simulink model "online_fuzz_clus"  (Simulink 7.7)
settings: Solver=ode4  StartTime=0.0  StopTime=10.0  FixedStep=0.01  RelTol=1e-3
undefined symbols (not defined in the file or in its folder): ali_veh_acc, ali_veh_spd, ali_veh_spdacc
settings Model: Creator=ali  LastModifiedBy=ali

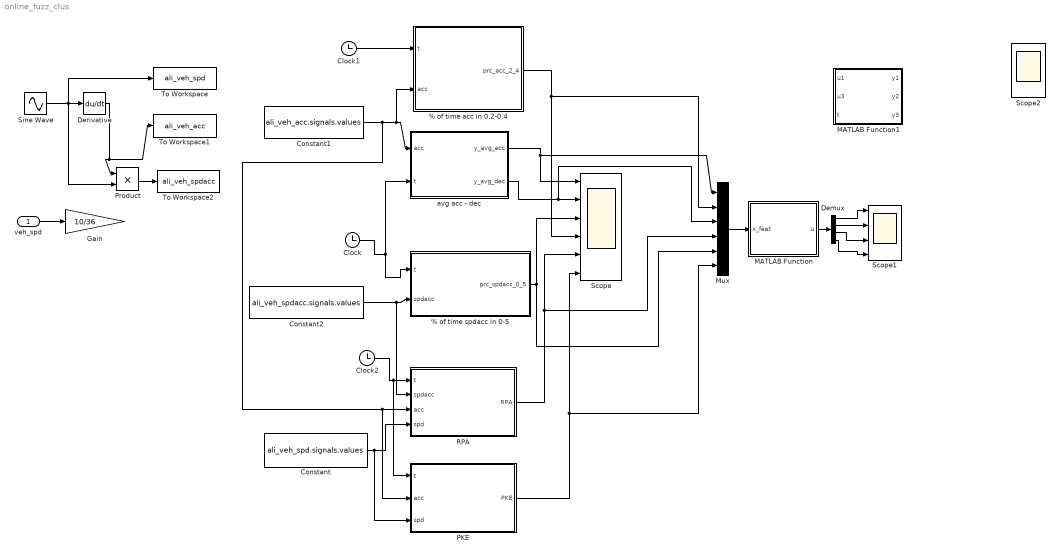
== system online_fuzz_clus ==
  veh_spd : Inport
  % of time acc in 0.2-0.4 : Stateflow chart  TreatAsAtomicUnit=on
  % of time spdacc in 0-5 : Stateflow chart  TreatAsAtomicUnit=on
  Clock : Clock
      settings: Decimation=10
  Clock1 : Clock
      settings: Decimation=10
  Clock2 : Clock
      settings: Decimation=10
  Constant : Constant  Value=ali_veh_spd.signals.values
  Constant1 : Constant  Value=ali_veh_acc.signals.values
  Constant2 : Constant  Value=ali_veh_spdacc.signals.values
  Demux : Demux
  Derivative : Derivative
  Gain : Gain  Gain=10/36
  MATLAB Function : Stateflow chart  TreatAsAtomicUnit=on
  MATLAB Function1 : Stateflow chart  TreatAsAtomicUnit=on
  Mux : Mux  Inputs=6
  PKE : Stateflow chart  TreatAsAtomicUnit=on
  Product : Product  RndMeth=Zero
  RPA : Stateflow chart  TreatAsAtomicUnit=on
  Scope : Scope  NumInputPorts=6
      settings: YMin=-5~-5~-5~-5~-5~-5  YMax=5~5~5~5~5~5
  Scope1 : Scope  NumInputPorts=4
      settings: YMin=-5~-5~-5~-5  YMax=5~5~5~5
  Scope2 : Scope  NumInputPorts=4
      settings: YMin=-5~-5~-5~-5  YMax=5~5~5~5  SaveName=ScopeData2
  Sine Wave : Sin  SampleTime=0
  To Workspace : ToWorkspace  VariableName=ali_veh_spd  SampleTime=-1  SaveFormat=Structure With Time
  To Workspace1 : ToWorkspace  VariableName=ali_veh_acc  SampleTime=-1  SaveFormat=Structure With Time
  To Workspace2 : ToWorkspace  VariableName=ali_veh_spdacc  SampleTime=-1  SaveFormat=Structure With Time
  avg acc - dec : Stateflow chart  TreatAsAtomicUnit=on
  wires:
  Sine Wave/1 -> Derivative/1, To Workspace/1, Product/2
  Derivative/1 -> To Workspace1/1, Product/1
  Clock/1 -> % of time spdacc in 0-5/1(t), avg acc - dec/2(t)
  Product/1 -> To Workspace2/1
  Constant2/1 -> % of time spdacc in 0-5/2(spdacc), RPA/2(spdacc)
  Constant1/1 -> avg acc - dec/1(acc), % of time acc in 0.2-0.4/2(acc), RPA/3(acc), PKE/2(acc)
  avg acc - dec/1(y_avg_acc) -> Scope/1, Mux/1
  avg acc - dec/2(y_avg_dec) -> Scope/2, Mux/3
  % of time spdacc in 0-5/1(prc_spdacc_0_5) -> Scope/3, Mux/5
  Clock1/1 -> % of time acc in 0.2-0.4/1(t)
  % of time acc in 0.2-0.4/1(prc_acc_2_4) -> Scope/4, Mux/2
  Clock2/1 -> RPA/1(t), PKE/1(t)
  Constant/1 -> PKE/3(spd), RPA/4(spd)
  RPA/1(RPA) -> Scope/5, Mux/4
  PKE/1(PKE) -> Scope/6, Mux/6
  veh_spd/1 -> Gain/1
  Mux/1 -> MATLAB Function/1(x_feat)
  MATLAB Function/1(u) -> Demux/1
  Demux/1 -> Scope1/1
  Demux/2 -> Scope1/2
  Demux/4 -> Scope1/4
  Demux/3 -> Scope1/3

== matlab function avg acc - dec ==
  data: y_avg_acc output double; acc input double; t input double; y_avg_dec output double
function [y_avg_acc,y_avg_dec] = fcn(acc,t)
k=round((t*100)+1);
sum_acc=0;sum_dec=0;
num_acc=0;num_dec=0;
y_avg_acc=0;y_avg_dec=0;
if t>2
    for i=k-200:k
        if acc(i)>0
            sum_acc=sum_acc+acc(i);
            num_acc=num_acc+1;
        end
        if acc(i)<0
            sum_dec=sum_dec+acc(i);
            num_dec=num_dec+1;
        end
    end
    y_avg_acc=sum_acc/num_acc;
    y_avg_dec=sum_dec/num_dec;
end
end

== matlab function % of time spdacc in 0-5 ==
  data: prc_spdacc_0_5 output double; t input double; spdacc input double
function prc_spdacc_0_5 = fcn(t,spdacc)
k=round((t*100)+1);
num=0;
if t>2
    for i=k-200:k
        if spdacc(i)<5 && spdacc(i)>0
            num=num+1;
        end
    end
end
prc_spdacc_0_5=num/200;
end

== matlab function % of time acc in 0.2-0.4 ==
  data: prc_acc_2_4 output double; t input double; acc input double
function prc_acc_2_4 = fcn(t,acc)
k=round((t*100)+1);
num=0;
if t>2
    for i=k-200:k
        if acc(i)<0.4 && acc(i)>0.2
            num=num+1;
        end
    end
end
prc_acc_2_4=num/200;
end

== matlab function RPA ==
  data: RPA output double; t input double; spdacc input double; acc input double; spd input double
function RPA = fcn(t,spdacc,acc,spd)
k=round((t*100)+1);
sum=0;dist=0;
RPA=0;
if t>2
    for i=k-200:k
        if acc(i)>0
            sum=sum+(0.5*(spdacc(i-1)+spdacc(i)));
            dist=dist+(0.01*spd(i));
        end
    end
    RPA=sum/dist;
end
end

== matlab function PKE ==
  data: PKE output double; t input double; acc input double; spd input double
function PKE = fcn(t,acc,spd)
k=round((t*100)+1);
sum=0;dist=0;
PKE=0;
if t>2
    for i=k-200:k
        if acc(i)>0
            sum=sum+((spd(i)^2 - spd(i-1)^2));
            dist=dist+(0.01*spd(i));
        end
    end
    PKE=sum/dist;
end
end

== matlab function MATLAB Function ==
  data: x_feat input double; u output double; teta parameter double
function u = fcn(x_feat, teta)
dist1=zeros(4,1);u=zeros(4,1);
p=4;q=2;dist2=zeros(4,1);
for j=1:4
    num=0;
    for e=1:6
        num=num+1;
        dist1(j)=dist1(j)+(((x_feat(e)-teta(e,j))/teta(e,j))^p);
    end
    dist2(j)=(dist1(j))^(1/p);
end
for k=1:4
    den=0;
    for t=1:4
        den=den+((dist2(k)/dist2(t))^(1/(q-1)));
    end
    u(k)=1/(den);
end
end

== matlab function MATLAB Function1 ==
  data: u1 input double; y1 output double; u2 parameter double; u3 input double; t input double; y2 output double; y3 output double
function [y1,y2,y3] = fcn(u1,u2,u3,t)
k=round((t*100)+1);
y1=u1(k);
y2=u2(k);
y3=u3(k);
end
